simulink model "Ejercicio2_TP_Control_PID"  (R2020a)
settings: Solver=VariableStepAuto  StartTime=0.0  StopTime=25.0  RelTol=1e-3
PreLoadFcn:
  | constantes_ej2
values from neighbouring files (symbols this model uses):
  a = 200    [Ejercicio4_Control_PID.m]    (also in constantes_ej1.m = 10000; constantes_ej2.m = 10000; constantes_ej3.m = 10000)
  b = 10000    [Ejercicio4_Control_PID.m]    (also in constantes_ej1.m = 200; constantes_ej2.m = 200; constantes_ej3.m = 200)
  g = 9.82    [Ejercicio4_Control_PID.m]    (also in constantes_ej1.m; constantes_ej2.m; constantes_ej3.m)
  kp = double(subs(kp_solu, [m_s, a_s, b_s, p_place_s], [m, a, b, p_place]))    [Ejercicio4_Control_PID.m]    (also in constantes_ej2.m = 1; constantes_ej3.m = 1)
  m = 1000    [Ejercicio4_Control_PID.m]    (also in constantes_ej1.m = 1500; constantes_ej2.m = 1500; constantes_ej3.m = 1500)
settings Model: Creator=Tomas  LastModifiedBy=Tomas

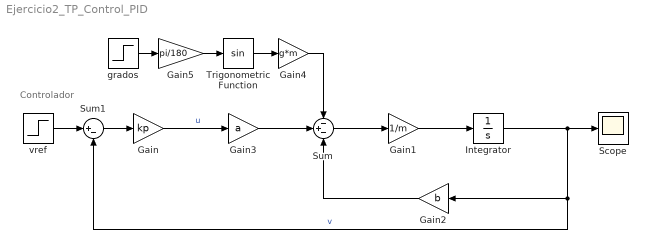
== system Ejercicio2_TP_Control_PID ==
  note: Controlador
  Gain : Gain  Gain=kp
  Gain1 : Gain  Gain=1/m
  Gain2 : Gain  Gain=b
  Gain3 : Gain  Gain=a
  Gain4 : Gain  Gain=g*m
  Gain5 : Gain  Gain=pi/180
  Integrator : Integrator  InitialCondition=25
  Scope : Scope
  Sum : Sum  Inputs=-+-
  Sum1 : Sum  Inputs=|+-
  Trigonometric Function : Trigonometry
  grados : Step  Time=20  After=0  SampleTime=0
  vref : Step  Time=10  Before=25  After=30  SampleTime=0
  wires:
  vref/1 -> Sum1/1
  Sum/1 -> Gain1/1
  Gain1/1 -> Integrator/1
  Integrator/1 -> Sum1/2, Gain2/1, Scope/1  "v"
  Sum1/1 -> Gain/1
  Gain2/1 -> Sum/3
  Gain3/1 -> Sum/2
  Trigonometric Function/1 -> Gain4/1
  grados/1 -> Gain5/1
  Gain5/1 -> Trigonometric Function/1
  Gain/1 -> Gain3/1  "u"
  Gain4/1 -> Sum/1
